simulink model "dynamic_bicycle2"  (R2019a)
settings: Solver=VariableStepAuto  StartTime=0.0  StopTime=1  RelTol=1e-3
values from neighbouring files (symbols this model uses):
  cornering_stiffness_front = 10000    [config_dynamic_bicycle.m]
  cornering_stiffness_rear = 10000    [config_dynamic_bicycle.m]
  init_states = [0,0,0,0,0,0,0]    [config_dynamic_bicycle.m]
  length_front = 1    [config_dynamic_bicycle.m]
  length_rear = 1    [config_dynamic_bicycle.m]
  mass = 200    [config_dynamic_bicycle.m]
  yaw_inertia = 50    [config_dynamic_bicycle.m]
libraries: simulink x2, simulink_extras x1
settings Model: Creator=jacoboffersen  LastModifiedBy=jacoboffersen

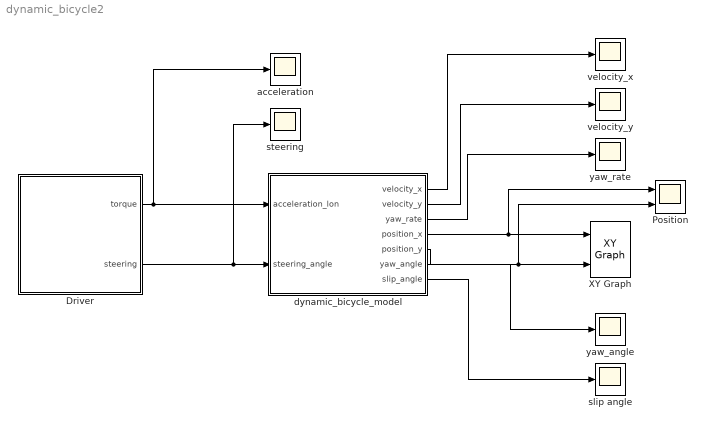
== system dynamic_bicycle2 ==
  Driver : Subsystem
  Position : Scope  NumInputPorts=2
  XY Graph : simulink/Sinks/XY Graph  xmin=-200  xmax=200  ymin=-200  ymax=200  st=-1
  acceleration : Scope
  "dynamic_bicycle_model " : Subsystem
  slip angle : Scope
  steering : Scope
  velocity_x : Scope
  velocity_y : Scope
  yaw_angle : Scope
  yaw_rate : Scope
  wires:
  Driver/2(steering) -> steering/1, "dynamic_bicycle_model "/2(steering_angle)
  Driver/1(torque) -> acceleration/1, "dynamic_bicycle_model "/1(acceleration_lon)
  "dynamic_bicycle_model "/4(position_x) -> Position/1, XY Graph/1
  "dynamic_bicycle_model "/5(position_y) -> Position/2, XY Graph/2
  "dynamic_bicycle_model "/6(yaw_angle) -> yaw_angle/1
  "dynamic_bicycle_model "/3(yaw_rate) -> yaw_rate/1
  "dynamic_bicycle_model "/2(velocity_y) -> velocity_y/1
  "dynamic_bicycle_model "/1(velocity_x) -> velocity_x/1
  "dynamic_bicycle_model "/7(slip_angle) -> slip angle/1

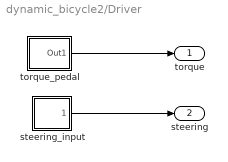
== system dynamic_bicycle2/Driver ==
  steering_input : Subsystem
  torque_pedal : Subsystem
  torque : Outport
  steering : Outport  Port=2
  wires:
  torque_pedal/1(Out1) -> torque/1
  steering_input/1(Out1) -> steering/1

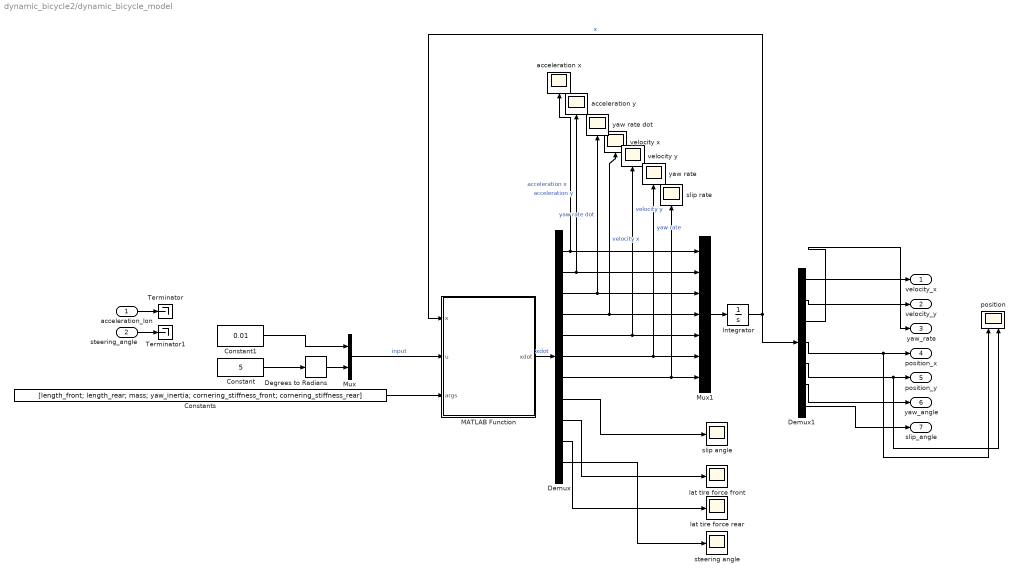
== system dynamic_bicycle2/dynamic_bicycle_model  ==
  acceleration_lon : Inport
  steering_angle : Inport  Port=2
  Constant : Constant  Value=5
  Constant1 : Constant  Value=0.01
  Constants : Constant  Value=[length_front; length_rear; mass; yaw_inertia; cornering_stiffness_front; cornering_stiffness_rear]
  Degrees to Radians : simulink_extras/Transformations/Degrees to Radians
  Demux : Demux  Outputs=11
  Demux1 : Demux  Outputs=7
  Integrator : Integrator  InitialCondition=init_states
  MATLAB Function : MATLAB Function  TreatAsAtomicUnit=on
  Mux : Mux  Inputs=2
  Mux1 : Mux  Inputs=7
  Terminator : Terminator
  Terminator1 : Terminator
  acceleration x : Scope
  acceleration y : Scope
  lat tire force front : Scope
  lat tire force rear : Scope
  position : Scope  NumInputPorts=2
  slip angle : Scope
  slip rate : Scope
  steering angle : Scope
  velocity x : Scope
  velocity y : Scope
  yaw rate : Scope
  yaw rate dot : Scope
  velocity_x : Outport
  velocity_y : Outport  Port=2
  yaw_rate : Outport  Port=3
  position_x : Outport  Port=4
  position_y : Outport  Port=5
  yaw_angle : Outport  Port=6
  slip_angle : Outport  Port=7
  wires:
  Mux/1 -> MATLAB Function/2(u)  "input"
  Constants/1 -> MATLAB Function/3(args)
  Integrator/1 -> Demux1/1, MATLAB Function/1(x)  "x"
  Demux1/2 -> velocity_y/1
  Demux1/1 -> velocity_x/1
  Demux1/3 -> yaw_rate/1
  Demux1/5 -> position/2, position_y/1
  Demux1/4 -> position/1, position_x/1
  Demux1/6 -> yaw_angle/1
  Mux1/1 -> Integrator/1
  MATLAB Function/1(xdot) -> Demux/1  "xdot"
  Demux/6 -> yaw rate/1, Mux1/6  "yaw rate"
  Demux/5 -> velocity y/1, Mux1/5  "velocity y"
  Demux/4 -> Mux1/4, velocity x/1  "velocity x"
  Demux/3 -> yaw rate dot/1, Mux1/3  "yaw rate dot"
  Demux/2 -> acceleration y/1, Mux1/2  "acceleration y"
  Demux/1 -> acceleration x/1, Mux1/1  "acceleration x"
  Constant1/1 -> Mux/1
  Degrees to Radians/1 -> Mux/2
  Constant/1 -> Degrees to Radians/1
  Demux/7 -> slip rate/1, Mux1/7
  Demux/8 -> slip angle/1
  Demux/9 -> lat tire force front/1
  Demux/10 -> lat tire force rear/1
  Demux/11 -> steering angle/1
  Demux1/7 -> slip_angle/1
  acceleration_lon/1 -> Terminator/1
  steering_angle/1 -> Terminator1/1

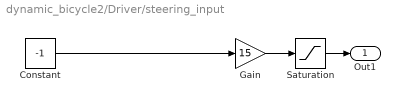
== system dynamic_bicycle2/Driver/steering_input ==
  Constant : Constant  Value=-1
  Gain : Gain  Gain=15
  Saturation : Saturate  UpperLimit=30  LowerLimit=-30
  Out1 : Outport
  wires:
  Saturation/1 -> Out1/1
  Gain/1 -> Saturation/1
  Constant/1 -> Gain/1

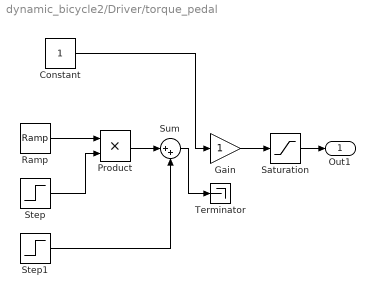
== system dynamic_bicycle2/Driver/torque_pedal ==
  Constant : Constant
  Gain : Gain
  Product : Product
  Ramp : simulink/Sources/Ramp  slope=1  start=1  InitialOutput=0
  Saturation : Saturate  UpperLimit=30  LowerLimit=-30
  Step : Step  Time=5  Before=1  After=0  SampleTime=0
  Step1 : Step  Time=5  After=0  SampleTime=0
  Sum : Sum  Inputs=|++
  Terminator : Terminator
  Out1 : Outport
  wires:
  Saturation/1 -> Out1/1
  Gain/1 -> Saturation/1
  Ramp/1 -> Product/1
  Step/1 -> Product/2
  Product/1 -> Sum/1
  Constant/1 -> Gain/1
  Step1/1 -> Sum/2
  Sum/1 -> Terminator/1

== matlab function dynamic_bicycle2/dynamic_bicycle_model /MATLAB Function ==
  data: x input; xdot output; u input; args input
function xdot = fcn(x, u, args)

velocity_x = x(1); % x velocity
velocity_y = x(2); % y velocity
yaw_rate   = x(3); % Yaw rate
position_x = x(4);
position_y = x(5);
yaw_angle  = x(6);
slip_angle = x(7);

acceleration_x  = u(1); % 
steering_angle  = u(2); % Steering angle

length_front              = args(1); % Length from front axle to CG
length_rear               = args(2); % Length from rear  axle to CG
mass                      = args(3);
yaw_inertia               = args(4);
cornering_stiffness_front = args(5);
cornering_stiffness_rear  = args(6);

% velocity = velocity_x + velocity_y;

% Tire forces
if(velocity_x > 0.001)
    lat_tire_force_front = cornering_stiffness_front*(steering_angle - slip_angle- (length_front*yaw_rate)/velocity_x);
    lat_tire_force_rear = cornering_stiffness_rear*(-slip_angle + (length_rear*yaw_rate)/velocity_x);
else
    lat_tire_force_front = cornering_stiffness_front*(steering_angle - slip_angle- (length_front*yaw_rate)/0.001);
    lat_tire_force_rear = cornering_stiffness_rear*(-slip_angle + (length_rear*yaw_rate)/0.001);
end



% SLIP RATE
% 3
if(velocity_x > 0.001)
    slip_rate_1 = cornering_stiffness_front/(mass*velocity_x)*(lat_tire_force_front);
    slip_rate_2 = cornering_stiffness_rear/(mass*velocity_x)*(lat_tire_force_rear);
%     slip_rate = -yaw_rate + slip_rate_1 + slip_rate_2;
else
   slip_rate_1 = cornering_stiffness_front/(mass*0.001)*(lat_tire_force_front);
    slip_rate_2 = cornering_stiffness_rear/(mass*0.001)*(lat_tire_force_rear);
end
slip_rate = -yaw_rate + slip_rate_1 + slip_rate_2;
% 2
% if(velocity > 0.001)
%     slip_rate_1= -(cornering_stiffness_rear+cornering_stiffness_front)/(mass*velocity)*steering_angle;
%     slip_rate_2 = ((cornering_stiffness_rear*length_rear-cornering_stiffness_front*length_front)/(mass*velocity) - 1);
%     slip_rate_3 = yaw_rate+cornering_stiffness_front/(mass*velocity)*steering_angle;
%     slip_rate = slip_rate_1 + slip_rate_2 * slip_rate_3;
% else
%     slip_rate = 0;
% end
% 1
% slip_rate = -(cornering_stiffness_rear+cornering_stiffness_front)/(mass*velocity)*steering_angle+...
%             ((cornering_stiffness_rear*length_rear-cornering_stiffness_front*length_front)/(mass*velocity) - 1)*...
%             yaw_rate+cornering_stiffness_front/(mass*velocity)*steering_angle;


% YAW RATE
% 3
yaw_rate_dot1 = ((length_front*cornering_stiffness_front)/yaw_inertia)*(lat_tire_force_front);
yaw_rate_dot2 = ((length_rear*cornering_stiffness_rear)/yaw_inertia)*(lat_tire_force_rear);
yaw_rate_dot = yaw_rate_dot1 - yaw_rate_dot2;
% 2
% yaw_rate_dot1 = (cornering_stiffness_rear*length_rear - cornering_stiffness_front*length_front)/(yaw_inertia)*steering_angle;
% if(velocity > 0.001)
%     yaw_rate_dot2 = (cornering_stiffness_rear*length_rear^2 + cornering_stiffness_front*length_front^2)/(yaw_inertia*velocity)*yaw_rate;
% else
%     yaw_rate_dot2 = 0;
% end
% yaw_rate_dot3 = (cornering_stiffness_front*length_front)/(yaw_inertia)*steering_angle;
% yaw_rate_dot = yaw_rate_dot1 - yaw_rate_dot2 + yaw_rate_dot3;
% 1
% yaw_rate_dot =  (cornering_stiffness_rear*length_rear - cornering_stiffness_front*length_front)/(yaw_inertia)*steering_angle-...
%                 (cornering_stiffness_rear*length_rear^2 + cornering_stiffness_front*length_front^2)/(yaw_inertia*velocity)*yaw_rate +...
%                 (cornering_stiffness_front*length_front)/yaw_inertia*steering_angle;




acceleration_y = velocity_x*slip_rate + velocity_y*yaw_rate;
            
xdot = [acceleration_x; 
        acceleration_y; 
        yaw_rate_dot; 
        velocity_x; 
        velocity_y; 
        yaw_rate; 
        slip_rate;
        slip_angle;
        lat_tire_force_front;
        lat_tire_force_rear;
        steering_angle];
